simulink library "dlbsBlockConcatenate"  (R2025b)
settings: Solver=VariableStepAuto  StartTime=0.0  StopTime=10.0  RelTol=1e-3
libraries: dlbsBlockInsertGradientGF x9, dlbsBlockParametrizedSelector x9, dlbsBlockExtractGradientGF x3
settings Model: Creator=lt6037  LastModifiedBy=lt6037

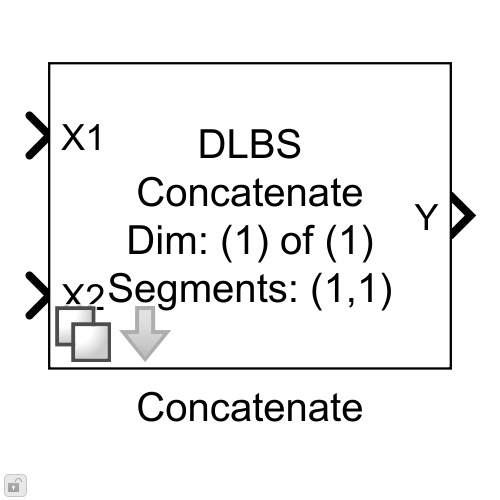
[thumbnail: Simulink's stored preview of the top-level diagram]
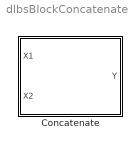
== system dlbsBlockConcatenate ==
  Concatenate : Subsystem  Variant=on  mask{n_out=2, all_dims=1, dim=1, s1=1, s2=1, s3=1, s4=1}
      mask prompts: n_out "Number of Inputs"; all_dims "Number of Dimensions"; dim "Working Dimension"; s1 "Length of Slice 1"; s2 "Length of Slice 2"; s3 "Length of Slice 3"; s4 "Length of Slice 4"
      mask help:
      | Concatenates multiple input tensors along a selected working dimension. The user must specify slice lengths for each active input, because these lengths are required to split the output gradient back to the corresponding input gradients.
      | The last tensor dimension must not be of size 1. If the last dimension would be 1, reduce ALL_DIMS by 1 and omit that trailing singleton dimension. This avoids Simulink implicitly dropping a singleton final dimension.
      mask Help: web("dlbsHelpBlockConcatenate.html")
      mask DialogControl Container3 Prompt: Last Indecies of Slices
      mask Display:
      | m = Simulink.Mask.get(gcb);
      | dim = m.getParameter("dim").Value;
      | all_dims = m.getParameter("all_dims").Value;
      | n_out = str2double(m.getParameter("n_out").Value);
      | 
      | lines = string.empty;
      | 
      | lines(end+1) = "DLBS";
      | lines(end+1) = "Concatenate";
      | lines(end+1) = sprintf("Dim: (%s) of (%s)",dim, all_dims);
      | 
      | for n = 1:n_out
      |     s(n) = string(m.getParameter(sprintf("s%d",n)).Value);
      | end
      | 
      | lines(end+1) = sprintf("Segments: (%s)", strjoin(s,","));
      | 
      | disp(strjoin(lines,"\n"));

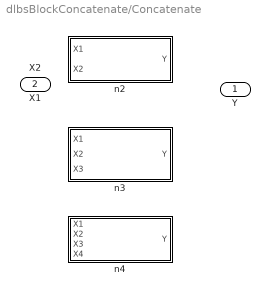
== system dlbsBlockConcatenate/Concatenate ==
  X1 : Inport
  X2 : Inport  Port=2
  n2 : Subsystem  VariantControl=n_out==2
  n3 : Subsystem  VariantControl=n_out==3
  n4 : Subsystem  VariantControl=n_out==4
  Y : Outport

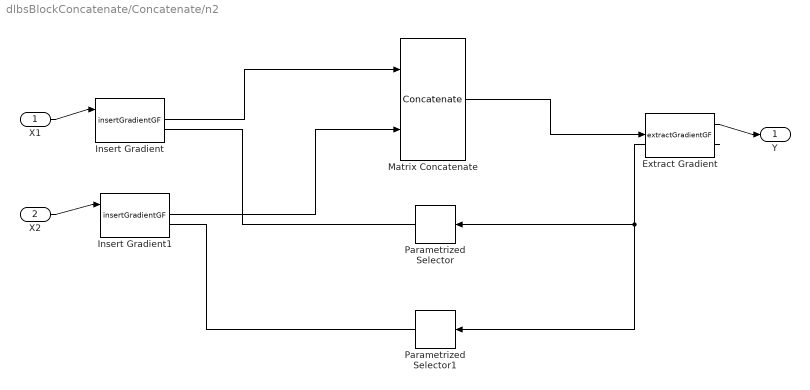
== system dlbsBlockConcatenate/Concatenate/n2 ==
  X1 : Inport
  X2 : Inport  Port=2
  Extract Gradient : dlbsBlockExtractGradientGF/extractGradientGF
  Insert Gradient : dlbsBlockInsertGradientGF/insertGradientGF
  Insert Gradient1 : dlbsBlockInsertGradientGF/insertGradientGF
  Matrix Concatenate : Concatenate  Mode=Multidimensional array  ConcatenateDimension=dim
  Parametrized Selector : dlbsBlockParametrizedSelector/Parametrized Selector  all_dims=all_dims  dim=dim  idx1=1  idx2=s1
  Parametrized Selector1 : dlbsBlockParametrizedSelector/Parametrized Selector  all_dims=all_dims  dim=dim  idx1=s1+1  idx2=s1+s2
  Y : Outport
  wires:
  X1/1 -> Insert Gradient/1
  Extract Gradient/1 -> Y/1
  X2/1 -> Insert Gradient1/1
  Insert Gradient/1 -> Matrix Concatenate/1
  Insert Gradient1/1 -> Matrix Concatenate/2
  Matrix Concatenate/1 -> Extract Gradient/1
  Extract Gradient/2 -> Parametrized Selector1/1, Parametrized Selector/1
  Parametrized Selector/1 -> Insert Gradient/2
  Parametrized Selector1/1 -> Insert Gradient1/2

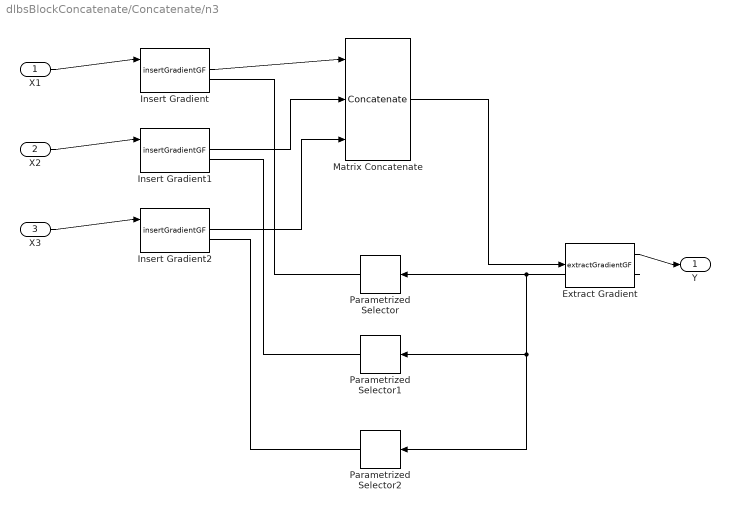
== system dlbsBlockConcatenate/Concatenate/n3 ==
  X1 : Inport
  X2 : Inport  Port=2
  X3 : Inport  Port=3
  Extract Gradient : dlbsBlockExtractGradientGF/extractGradientGF
  Insert Gradient : dlbsBlockInsertGradientGF/insertGradientGF
  Insert Gradient1 : dlbsBlockInsertGradientGF/insertGradientGF
  Insert Gradient2 : dlbsBlockInsertGradientGF/insertGradientGF
  Matrix Concatenate : Concatenate  NumInputs=3  Mode=Multidimensional array  ConcatenateDimension=dim
  Parametrized Selector : dlbsBlockParametrizedSelector/Parametrized Selector  all_dims=all_dims  dim=dim  idx1=1  idx2=1+s1-1
  Parametrized Selector1 : dlbsBlockParametrizedSelector/Parametrized Selector  all_dims=all_dims  dim=dim  idx1=s1+1  idx2=s1+s2
  Parametrized Selector2 : dlbsBlockParametrizedSelector/Parametrized Selector  all_dims=all_dims  dim=dim  idx1=s1+s2+1  idx2=s1+s2+s3
  Y : Outport
  wires:
  X1/1 -> Insert Gradient/1
  X2/1 -> Insert Gradient1/1
  X3/1 -> Insert Gradient2/1
  Extract Gradient/1 -> Y/1
  Insert Gradient/1 -> Matrix Concatenate/1
  Insert Gradient1/1 -> Matrix Concatenate/2
  Insert Gradient2/1 -> Matrix Concatenate/3
  Parametrized Selector/1 -> Insert Gradient/2
  Parametrized Selector1/1 -> Insert Gradient1/2
  Parametrized Selector2/1 -> Insert Gradient2/2
  Extract Gradient/2 -> Parametrized Selector/1, Parametrized Selector2/1, Parametrized Selector1/1
  Matrix Concatenate/1 -> Extract Gradient/1

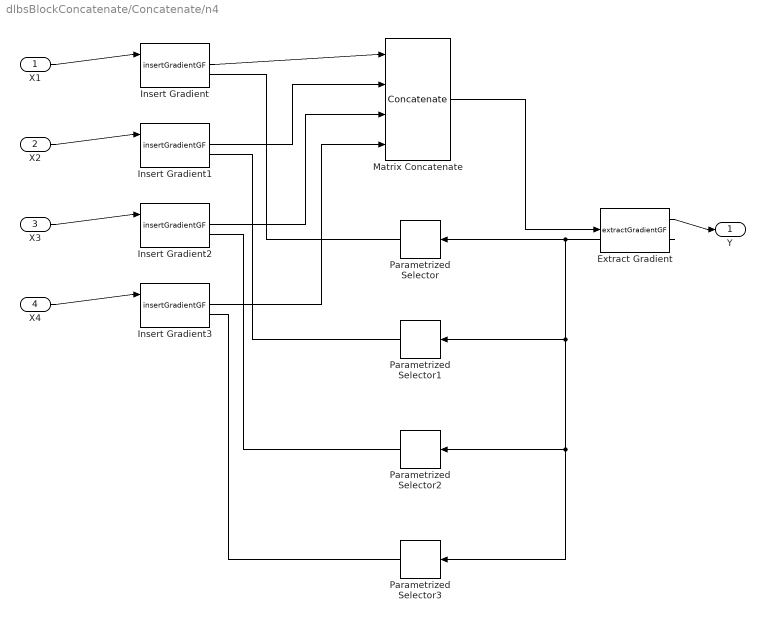
== system dlbsBlockConcatenate/Concatenate/n4 ==
  X1 : Inport
  X2 : Inport  Port=2
  X3 : Inport  Port=3
  X4 : Inport  Port=4
  Extract Gradient : dlbsBlockExtractGradientGF/extractGradientGF
  Insert Gradient{,1..3} (4 alike) : dlbsBlockInsertGradientGF/insertGradientGF
  Matrix Concatenate : Concatenate  NumInputs=4  Mode=Multidimensional array  ConcatenateDimension=dim
  Parametrized Selector : dlbsBlockParametrizedSelector/Parametrized Selector  all_dims=all_dims  dim=dim  idx1=1  idx2=1+s1-1
  Parametrized Selector1 : dlbsBlockParametrizedSelector/Parametrized Selector  all_dims=all_dims  dim=dim  idx1=s1+1  idx2=s1+s2
  Parametrized Selector2 : dlbsBlockParametrizedSelector/Parametrized Selector  all_dims=all_dims  dim=dim  idx1=s1+s2+1  idx2=s1+s2+s3
  Parametrized Selector3 : dlbsBlockParametrizedSelector/Parametrized Selector  all_dims=all_dims  dim=dim  idx1=s1+s2+s3+1  idx2=s1+s2+s3+s4
  Y : Outport
  wires:
  Extract Gradient/1 -> Y/1
  X1/1 -> Insert Gradient/1
  X2/1 -> Insert Gradient1/1
  X3/1 -> Insert Gradient2/1
  X4/1 -> Insert Gradient3/1
  Insert Gradient/1 -> Matrix Concatenate/1
  Insert Gradient1/1 -> Matrix Concatenate/2
  Extract Gradient/2 -> Parametrized Selector/1, Parametrized Selector3/1, Parametrized Selector2/1, Parametrized Selector1/1
  Insert Gradient2/1 -> Matrix Concatenate/3
  Insert Gradient3/1 -> Matrix Concatenate/4
  Matrix Concatenate/1 -> Extract Gradient/1
  Parametrized Selector/1 -> Insert Gradient/2
  Parametrized Selector1/1 -> Insert Gradient1/2
  Parametrized Selector2/1 -> Insert Gradient2/2
  Parametrized Selector3/1 -> Insert Gradient3/2
